simulink model "adaptive_control"  (R2016a)
settings: Solver=VariableStepAuto  StartTime=0.0  StopTime=10.0  RelTol=1e-3
settings Model: Creator=Aniket  LastModifiedBy=Aniket

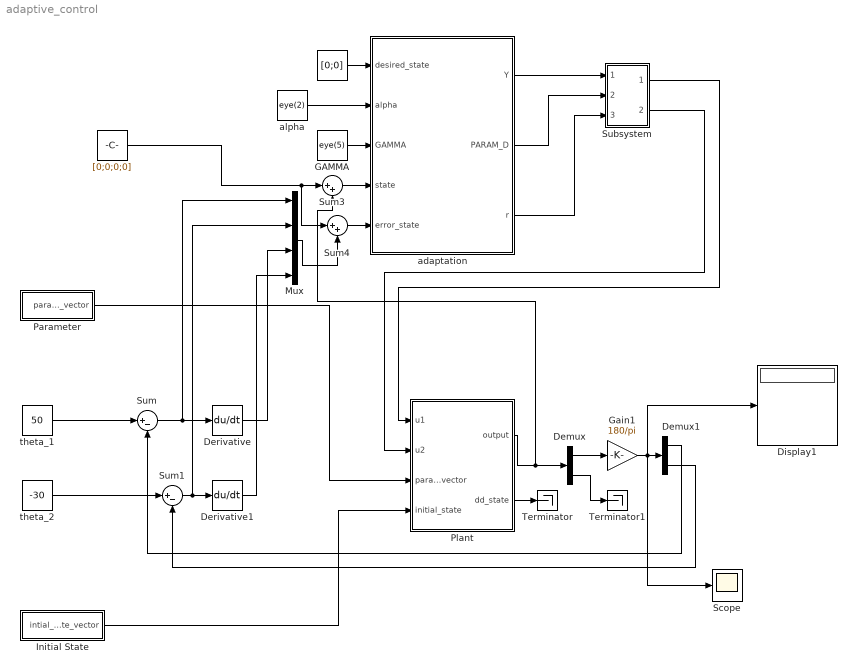
== system adaptive_control ==
  " " : Constant  Value=[0;0]
  "   " : Constant  Value=[0;0;0;0]
  Demux : Demux  Outputs=2
  Demux1 : Demux  Outputs=2
  Derivative : Derivative
  Derivative1 : Derivative
  Display1 : Display
  GAMMA : Constant  Value=eye(5)
  Gain1 : Gain  Gain=180/pi
  Initial State : Subsystem
  Mux : Mux
  Parameter : Subsystem
  Plant : Subsystem
  Scope : Scope
  Subsystem : Subsystem
  Sum : Sum  Inputs=|+-
  Sum1 : Sum  Inputs=|+-
  Sum3 : Sum  Inputs=|++
  Sum4 : Sum  Inputs=|++
  Terminator : Terminator
  Terminator1 : Terminator
  adaptation : MATLAB Function  TreatAsAtomicUnit=on
  alpha : Constant  Value=eye(2)
  theta_1 : Constant  Value=50
  theta_2 : Constant  Value=-30
  wires:
  " "/1 -> adaptation/1(desired_state)
  alpha/1 -> adaptation/2(alpha)
  GAMMA/1 -> adaptation/3(GAMMA)
  Plant/1(output) -> Sum3/2, Demux/1
  Demux/1 -> Gain1/1
  theta_1/1 -> Sum/1
  theta_2/1 -> Sum1/1
  Sum/1 -> Mux/1, Derivative/1
  Sum1/1 -> Mux/2, Derivative1/1
  Gain1/1 -> Display1/1, Scope/1, Demux1/1
  Demux1/1 -> Sum/2
  Demux1/2 -> Sum1/2
  Parameter/1("param_vector ") -> Plant/3(param_vector)
  Initial State/1(intial_state_vector) -> Plant/4(initial_state)
  Plant/2(dd_state) -> Terminator/1
  Demux/2 -> Terminator1/1
  Derivative/1 -> Mux/3
  Derivative1/1 -> Mux/4
  Sum3/1 -> adaptation/4(state)
  "   "/1 -> Sum4/1, Sum3/1
  Mux/1 -> Sum4/2
  Sum4/1 -> adaptation/5(error_state)
  adaptation/1(Y) -> Subsystem/1(In1)
  adaptation/2(PARAM_D) -> Subsystem/2(In2)
  adaptation/3(r) -> Subsystem/3(In3)
  Subsystem/1(Out1) -> Plant/1(u1)
  Subsystem/2(Out2) -> Plant/2(u2)

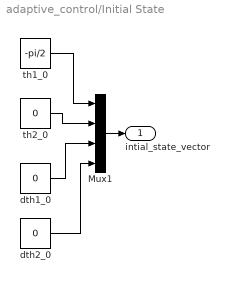
== system adaptive_control/Initial State ==
  Mux1 : Mux
  dth1_0 : Constant  Value=0
  dth2_0 : Constant  Value=0
  th1_0 : Constant  Value=-pi/2
  th2_0 : Constant  Value=0
  intial_state_vector : Outport
  wires:
  Mux1/1 -> intial_state_vector/1
  dth2_0/1 -> Mux1/4
  th1_0/1 -> Mux1/1
  dth1_0/1 -> Mux1/3
  th2_0/1 -> Mux1/2

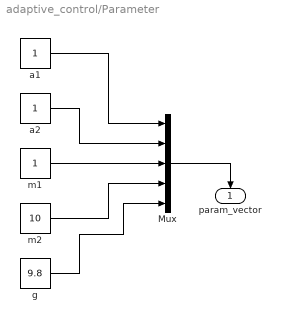
== system adaptive_control/Parameter ==
  Mux : Mux  Inputs=5
  "a1 " : Constant
  a2 : Constant
  g : Constant  Value=9.8
  m1 : Constant
  m2 : Constant  Value=10
  "param_vector " : Outport
  wires:
  m1/1 -> Mux/3
  Mux/1 -> "param_vector "/1
  g/1 -> Mux/5
  "a1 "/1 -> Mux/1
  m2/1 -> Mux/4
  a2/1 -> Mux/2

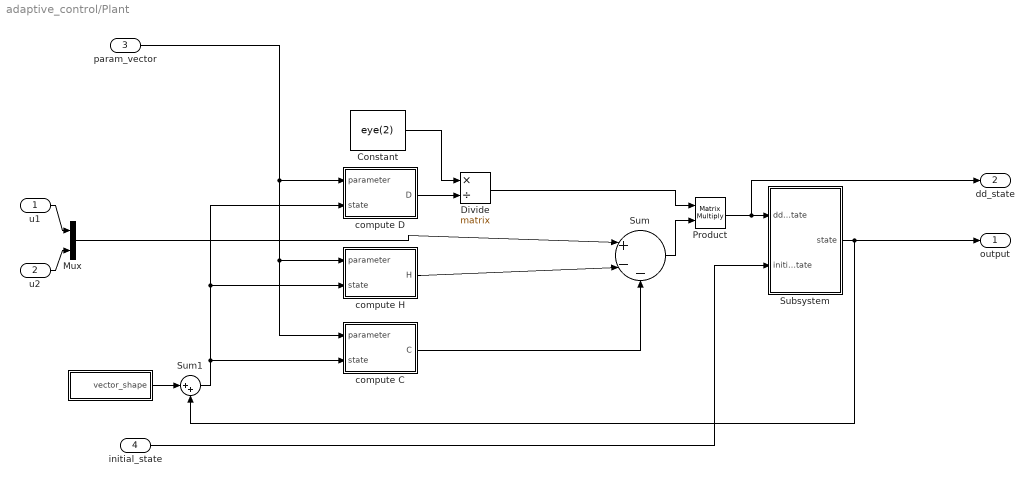
== system adaptive_control/Plant ==
  u1 : Inport
  u2 : Inport  Port=2
  param_vector : Inport  Port=3
  initial_state : Inport  Port=4
  "  " : Subsystem
  Constant : Constant  Value=eye(2)
  Divide : Product  Inputs=*/  Multiplication=Matrix(*)
  Mux : Mux  Inputs=2
  Product : Product  Multiplication=Matrix(*)
  Subsystem : Subsystem
  Sum : Sum  Inputs=|+--
  Sum1 : Sum  Inputs=|++
  compute C : MATLAB Function  TreatAsAtomicUnit=on
  compute D : MATLAB Function  TreatAsAtomicUnit=on
  compute H : MATLAB Function  TreatAsAtomicUnit=on
  output : Outport
  dd_state : Outport  Port=2
  wires:
  Sum/1 -> Product/2
  compute C/1(C) -> Sum/3
  Constant/1 -> Divide/1
  initial_state/1 -> Subsystem/2(initial_state)
  compute H/1(H) -> Sum/2
  compute D/1(D) -> Divide/2
  Mux/1 -> Sum/1
  param_vector/1 -> compute C/1(parameter), compute H/1(parameter), compute D/1(parameter)
  Product/1 -> dd_state/1, Subsystem/1(dd_state)
  Sum1/1 -> compute D/2(state), compute H/2(state), compute C/2(state)
  "  "/1(vector_shape) -> Sum1/1
  Divide/1 -> Product/1
  u1/1 -> Mux/1
  Subsystem/1(state) -> output/1, Sum1/2
  u2/1 -> Mux/2

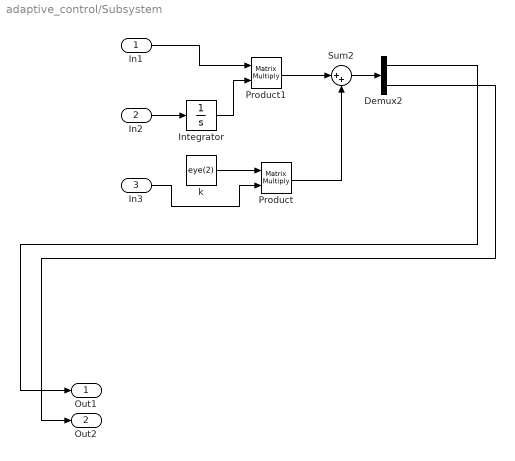
== system adaptive_control/Subsystem ==
  In1 : Inport
  In2 : Inport  Port=2
  In3 : Inport  Port=3
  Demux2 : Demux  Outputs=2
  Integrator : Integrator
  Product : Product  Multiplication=Matrix(*)
  Product1 : Product  Multiplication=Matrix(*)
  Sum2 : Sum  Inputs=|++
  k : Constant  Value=eye(2)
  Out1 : Outport
  Out2 : Outport  Port=2
  wires:
  In2/1 -> Integrator/1
  In3/1 -> Product/2
  Sum2/1 -> Demux2/1
  Product1/1 -> Sum2/1
  k/1 -> Product/1
  Integrator/1 -> Product1/2
  Demux2/2 -> Out2/1
  Demux2/1 -> Out1/1
  Product/1 -> Sum2/2
  In1/1 -> Product1/1

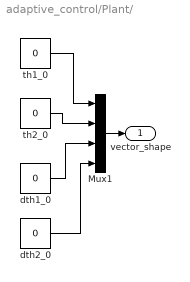
== system adaptive_control/Plant/   ==
  Mux1 : Mux
  dth1_0 : Constant  Value=0
  dth2_0 : Constant  Value=0
  th1_0 : Constant  Value=0
  th2_0 : Constant  Value=0
  vector_shape : Outport
  wires:
  th2_0/1 -> Mux1/2
  dth1_0/1 -> Mux1/3
  th1_0/1 -> Mux1/1
  dth2_0/1 -> Mux1/4
  Mux1/1 -> vector_shape/1

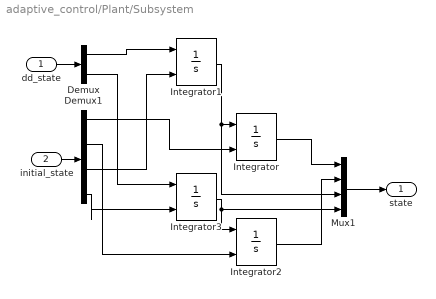
== system adaptive_control/Plant/Subsystem ==
  dd_state : Inport
  initial_state : Inport  Port=2
  Demux : Demux  Outputs=2
  Demux1 : Demux
  Integrator{,1..3} (4 alike) : Integrator  InitialConditionSource=external
  Mux1 : Mux
  state : Outport
  wires:
  initial_state/1 -> Demux1/1
  dd_state/1 -> Demux/1
  Integrator/1 -> Mux1/1
  Integrator2/1 -> Mux1/2
  Demux/1 -> Integrator1/1
  Demux/2 -> Integrator3/1
  Integrator1/1 -> Mux1/3, Integrator/1
  Integrator3/1 -> Mux1/4, Integrator2/1
  Demux1/3 -> Integrator1/2
  Demux1/4 -> Integrator3/2
  Mux1/1 -> state/1
  Demux1/2 -> Integrator2/2
  Demux1/1 -> Integrator/2

== matlab function adaptive_control/Plant/compute D ==
  data: parameter input; D output; state input
function D = D(parameter,state)
a1 = parameter(1);
a2 = parameter(2);
m1 = parameter(3);
m2 = parameter(4);
g = parameter(5);

if isempty(state)
    th1 = 0;
    th2 = 0;
    thd1 = 0;
    thd2 = 0;
else
    th1 = state(1);
    th2 = state(2);
    thd1 = state(3);
    thd2 = state(4);
end

D = [ (a1^2*m1)/3 + a1^2*m2 + (a2^2*m2)/3 + a1*a2*m2*cos(th2), (a2*m2*(2*a2 + 3*a1*cos(th2)))/6;
    (a2*m2*(2*a2 + 3*a1*cos(th2)))/6,                      (a2^2*m2)/3];

== matlab function adaptive_control/adaptation ==
  data: Y output; desired_state input; PARAM_D output; alpha input; GAMMA input; state input; error_state input; r output
function [Y,PARAM_D,r]= adaptation(desired_state,alpha,GAMMA,state,error_state)
 e = [error_state(1);error_state(2)];
 e_d = [error_state(3);error_state(4)];
 e1 = e(1); e2 = e(2);
 e1_d = e_d(1); e2_d = e_d(2);
 a1 = alpha(1);
 a2 = alpha(4);
 t1 = state(1);
 t2 = state(2);
 t1_d = state(3);
 t2_d = state(4);
 t1d_dd = desired_state(1);
 t2d_dd = desired_state(2);
 Y = [cos(t1) t1d_dd+a1*e1_d cos(t1+t2) (2*t1d_dd+t2d_dd+2*a1*e1_d+a2*e2_d)*cos(t2)-t2_d*(2*t1_d+t2_d)*sin(t2) t1d_dd+t2d_dd+a1*e1_d+a2*e2_d;
     0       0              cos(t1+t2) (t1d_dd+a1*e1_d)*cos(t2)+t1_d^2*sin(t2)                                t1d_dd+t2d_dd+a1*e1_d+a2*e2_d];
 r = e_d+alpha*e;
 PARAM_D = GAMMA*Y'*r;

== matlab function adaptive_control/Plant/compute C ==
  data: parameter input; C output; state input
function C = C(parameter,state)
a1 = parameter(1);
a2 = parameter(2);
m1 = parameter(3);
m2 = parameter(4);
g = parameter(5);
if isempty(state)
    th1 = 0;
    th2 = 0;
    thd1 = 0;
    thd2 = 0;
else
    th1 = state(1);
    th2 = state(2);
    thd1 = state(3);
    thd2 = state(4);
end
C = [(g*(a1*m1*cos(th1) + 2*a1*m2*cos(th1) + a2*m2*cos(th1 + th2)))/2;
                                       (a2*g*m2*cos(th1 + th2))/2];

== matlab function adaptive_control/Plant/compute H ==
  data: parameter input; H output; state input
function H = H(parameter,state)
a1 = parameter(1);
a2 = parameter(2);
m1 = parameter(3);
m2 = parameter(4);
g = parameter(5);

if isempty(state)
    th1 = 0;
    th2 = 0;
    thd1 = 0;
    thd2 = 0;
else
    th1 = state(1);
    th2 = state(2);
    thd1 = state(3);
    thd2 = state(4);
end
H = [ -(a1*a2*m2*thd2*sin(th2)*(2*thd1 + thd2))/2;
                (a1*a2*m2*thd1^2*sin(th2))/2];
